simulink model "lab2"  (R2016a)
settings: Solver=FixedStepDiscrete  StartTime=0.0  StopTime=inf  FixedStep=Ts  RelTol=1e-3
values from neighbouring files (symbols this model uses):
  feedback_gain = [0 0 0 0]    [setup_lab2.m]    (also in your_code.m = dlqr(Phi, Gam, Q1, Q2); your_code1.m = dlqr(d_sys.A, d_sys.B, Q1, Q2); your_code2.m = dlqr(Phi, Gam, Q1, Q2); your_code3.m = dlqr(Phi, Gam, Q1, Q2))
  integral_gain = 0    [setup_lab2.m]
undefined symbols (not defined in the file or in its folder): DiscIntNeverNeededParam
libraries: cstblocks x2, MinSegLibrary_M1V4 x2, simulink x1, dspsigops x1
settings Model: SimulationMode=external  ExtModeTrigDuration=2  Creator=Alec  LastModifiedBy=nilsv
settings DataIOCC: LimitDataPoints=on  SaveFormat=Array  SaveOutput=off  SignalLogging=off  DSMLogging=off  VisualizeSimOutput=off  SaveTime=off
settings OptimizationCC: PassReuseOutputArgsThreshold=0  ExpressionDepthLimit=2147483647  MaxStackSize=64
settings DebuggingCC: UnderspecifiedInitializationDetection=Classic  MergeDetectMultiDrivingBlocksExec=none  ParameterTunabilityLossMsg=error  UnconnectedInputMsg=none  UnconnectedOutputMsg=none  StateNameClashWarn=warning
settings HardwareCC: ProdBitPerInt=16  ProdBitPerPointer=16  ProdLargestAtomicFloat=None  ProdWordSize=8  ProdHWDeviceType=Atmel->AVR  UseEmbeddedCoderFeatures=off  UseSimulinkCoderFeatures=off
settings ModelReferenceCC: PropagateSignalLabelsOutOfModel=off
settings RTWCC: SystemTargetFile=ert.tlc  HardwareBoard=Arduino Mega 2560  TLCOptions=-aInlineSetEventsForThisBaseRateFcn=TLC_FALSE -aSuppressMultiTaskScheduler=TLC_FALSE -aRateBasedStepFcn=1  TemplateMakefile=ert_default_tmf  RTWVerbose=off  Toolchain=Arduino AVR v1.6.1  BuildConfiguration=Faster Runs
settings CodeAppCC: ForceParamTrailComments=on  OperatorAnnotations=on  MangleLength=10
settings ERTTargetCC: MultiwordLength=256  ERTCustomFileBanners=off  SupportContinuousTime=on  SupportNonInlinedSFcns=on  SupportVariableSizeSignals=on  ModelStepFunctionPrototypeControlCompliant=off  ExtMode=on  ExtModeTransport=3  ExtModeMexFile=ext_serial_win32_comm_rtt  ExtModeMexArgs=0 '/dev/ttyACM0' 115200  ERTSrcFileBannerTemplate=codertarget_code_template.cgt  ERTHdrFileBannerTemplate=codertarget_code_template.cgt  ERTDataSrcFileTemplate=codertarget_code_template.cgt  ERTDataHdrFileTemplate=codertarget_code_template.cgt
settings ConfigComp: CovEnableCumulative=off  CovSaveSingleToWorkspaceVar=off  CovSaveOutputData=off

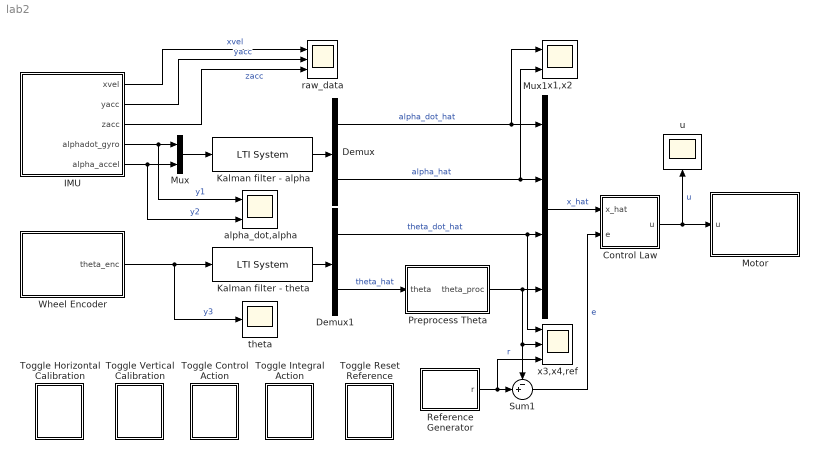
== system lab2 ==
  Control Law : Subsystem
  Demux : Demux  Outputs=2
  Demux1 : Demux  Outputs=2
  IMU : Subsystem
  Kalman filter - alpha : cstblocks/LTI System  sys=imu_kalman  IC=[]
  Kalman filter - theta : cstblocks/LTI System  sys=wheel_kalman  IC=[]
  Motor : Subsystem
  Mux : Mux  Inputs=2
  Mux1 : Mux
  Preprocess Theta : Subsystem
  Reference Generator : Subsystem  mask{amplitude_reference=0}
      mask prompts: amplitude_reference "Amplitude"
      mask DialogControl DescTextVar Prompt: Reference Generator. Please set the amplitude of the reference signal to follow.
      mask Display:
      | y = [-1,-1,-1,-1,-1,-1,-1,-1,-1,-0.6,-0.2,0.2,0.6,1,1,1,1,1,1,1,1,1,1,1,1,1,1,1,1,1,1,0.6,0.2,-0.2,-0.6,-1,-1,-1,-1,-1,-1,-1,-1,-1];
      | x = [-1,-0.96078,-0.92157,-0.88235,-0.84314,-0.80392,-0.76471,-0.72549,-0.68627,-0.56863,-0.52941,-0.4902,-0.45098,-0.33333,-0.29412,-0.2549,-0.21569,-0.17647,-0.13725,-0.098039,-0.058824,-0.019608,0.019608,0.058824,0.098039,0.13725,0.17647,0.21569,0.2549,0.29412,0.33333,0.45098,0.4902,0.52941,0.56863,0.68627,0.72549,0.76471,0.80392,0.84314,0.88235,0.92157,0.96078,1];
      | plot(x, y);
  Sum1 : Sum  Inputs=-+|
  Toggle Control Action : Subsystem  DialogController=hmiCreateDDGDialog  IsWebBlock=on  mask(MWDashboardBlock){webBlockId=64fc8a19-04bc-47ff-b6b8-cd18ab5ec033, webBlockType=toggleswitch, ShowInLibBrowser=on, ShowInitialText=on, HMISrcModelName=lab2}
      mask prompts: webBlockId "WebBlock Id"; webBlockType "WebBlock Type"; HMISrcModelName "Source Model"
      mask Help: helpview([docroot '/mapfiles/simulink.map'], 'hmi_toggle_switch')
      mask Display:
      | if strcmp(get_param(bdroot(gcb),'BlockDiagramType'), 'library')
      |     image([(matlabroot) '/toolbox/simulink/hmi/icons/ToggleSwitch.png']);
      | end
  Toggle Integral Action : Subsystem  DialogController=hmiCreateDDGDialog  IsWebBlock=on  mask(MWDashboardBlock){webBlockId=4f1e93d4-160d-4872-a41a-e243eeba8d4a, webBlockType=toggleswitch, ShowInLibBrowser=on, ShowInitialText=on, HMISrcModelName=lab2}
      mask prompts: webBlockId "WebBlock Id"; webBlockType "WebBlock Type"; HMISrcModelName "Source Model"
      mask Help: helpview([docroot '/mapfiles/simulink.map'], 'hmi_toggle_switch')
      mask Display:
      | if strcmp(get_param(bdroot(gcb),'BlockDiagramType'), 'library')
      |     image([(matlabroot) '/toolbox/simulink/hmi/icons/ToggleSwitch.png']);
      | end
  Toggle Reset Reference : Subsystem  DialogController=hmiCreateDDGDialog  IsWebBlock=on  mask(MWDashboardBlock){webBlockId=51dc4b42-a644-48db-9e68-323c48c3ab41, webBlockType=toggleswitch, ShowInLibBrowser=on, ShowInitialText=on, HMISrcModelName=lab2}
      mask prompts: webBlockId "WebBlock Id"; webBlockType "WebBlock Type"; HMISrcModelName "Source Model"
      mask Help: helpview([docroot '/mapfiles/simulink.map'], 'hmi_toggle_switch')
      mask Display:
      | if strcmp(get_param(bdroot(gcb),'BlockDiagramType'), 'library')
      |     image([(matlabroot) '/toolbox/simulink/hmi/icons/ToggleSwitch.png']);
      | end
  Toggle Horizontal Calibration : Subsystem  DialogController=hmiCreateDDGDialog  IsWebBlock=on  mask(MWDashboardBlock){webBlockId=eadab8c8-cd35-48e9-8b59-a5b0521da82c, webBlockType=toggleswitch, ShowInLibBrowser=on, ShowInitialText=on, HMISrcModelName=lab2}
      mask prompts: webBlockId "WebBlock Id"; webBlockType "WebBlock Type"; HMISrcModelName "Source Model"
      mask Help: helpview([docroot '/mapfiles/simulink.map'], 'hmi_toggle_switch')
      mask Display:
      | if strcmp(get_param(bdroot(gcb),'BlockDiagramType'), 'library')
      |     image([(matlabroot) '/toolbox/simulink/hmi/icons/ToggleSwitch.png']);
      | end
  Toggle Vertical Calibration : Subsystem  DialogController=hmiCreateDDGDialog  IsWebBlock=on  mask(MWDashboardBlock){webBlockId=45f31a6e-857f-48e6-b054-7e32dd315763, webBlockType=toggleswitch, ShowInLibBrowser=on, ShowInitialText=on, HMISrcModelName=lab2}
      mask prompts: webBlockId "WebBlock Id"; webBlockType "WebBlock Type"; HMISrcModelName "Source Model"
      mask Help: helpview([docroot '/mapfiles/simulink.map'], 'hmi_toggle_switch')
      mask Display:
      | if strcmp(get_param(bdroot(gcb),'BlockDiagramType'), 'library')
      |     image([(matlabroot) '/toolbox/simulink/hmi/icons/ToggleSwitch.png']);
      | end
  Wheel Encoder : Subsystem
  alpha_dot,alpha : Scope  NumInputPorts=2
  raw_data : Scope  NumInputPorts=3
  theta : Scope
  u : Scope
  x1,x2 : Scope  NumInputPorts=2
  x3,x4,ref : Scope  NumInputPorts=3
  wires:
  Mux/1 -> Kalman filter - alpha/1
  Demux/2 -> x1,x2/2, Mux1/2  "alpha_hat"
  Demux/1 -> x1,x2/1, Mux1/1  "alpha_dot_hat"
  Mux1/1 -> Control Law/1(x_hat)  "x_hat"
  Wheel Encoder/1(theta_enc) -> theta/1, Kalman filter - theta/1  "y3"
  Demux1/1 -> x3,x4,ref/1, Mux1/3  "theta_dot_hat"
  Demux1/2 -> Preprocess Theta/1(theta)  "theta_hat"
  Kalman filter - theta/1 -> Demux1/1
  Control Law/1(u) -> Motor/1(u), u/1  "u"
  IMU/5(alpha_accel) -> alpha_dot,alpha/2, Mux/2  "y2"
  IMU/4(alphadot_gyro) -> alpha_dot,alpha/1, Mux/1  "y1"
  Reference Generator/1(r) -> Sum1/2, x3,x4,ref/3  "r"
  Preprocess Theta/1(theta_proc) -> Mux1/4, Sum1/1, x3,x4,ref/2
  Kalman filter - alpha/1 -> Demux/1
  Sum1/1 -> Control Law/2(e)  "e"
  IMU/1(xvel) -> raw_data/1  "xvel"
  IMU/3(zacc) -> raw_data/3  "zacc"
  IMU/2(yacc) -> raw_data/2  "yacc"

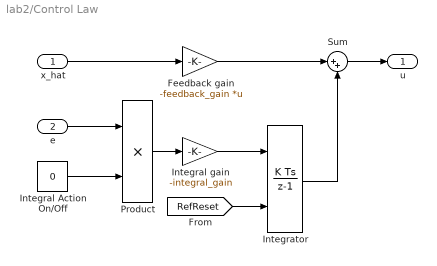
== system lab2/Control Law ==
  x_hat : Inport
  e : Inport  Port=2
  Feedback gain : Gain  Gain=-feedback_gain  Multiplication=Matrix(K*u)
  Integral Action On/Off : Constant  Value=0
  Integral gain : Gain  Gain=-integral_gain
  Integrator : DiscreteIntegrator  gainval=1  ExternalReset=either  InitialConditionSetting=State (most efficient)  SampleTime=-1  ICPrevOutput=DiscIntNeverNeededParam  ICPrevScaledInput=DiscIntNeverNeededParam
  Product : Product
  Sum : Sum  Inputs=|++
  u : Outport
  wires:
  Integral gain/1 -> Integrator/1
  x_hat/1 -> Feedback gain/1
  Feedback gain/1 -> Sum/1
  Sum/1 -> u/1
  Product/1 -> Integral gain/1
  e/1 -> Product/1
  Integral Action On/Off/1 -> Product/2
  Integrator/1 -> Sum/2
  [RefReset] -> Integrator/2

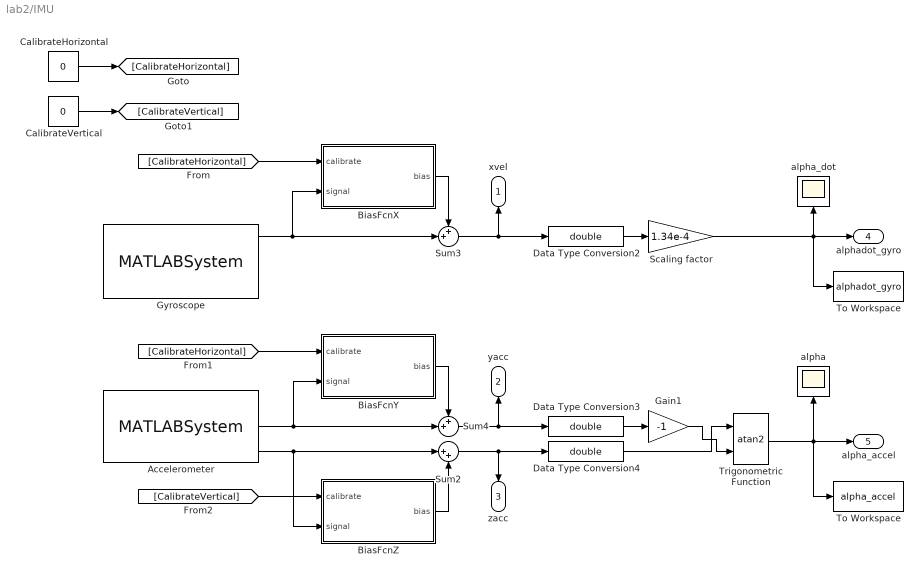
== system lab2/IMU ==
  " To Workspace " : ToWorkspace  VariableName=alpha_accel  SampleTime=-1
      settings: Save2DSignal=2-D array (concatenate along first dimension)
  Accelerometer : MATLABSystem  System=soMPU6050Accel  SimulateUsing=Code generation
      mask Type: soMPU6050Accel
      mask Display:
      | disp('soMPU6050Accel');
      | port_label('output',1,'xaccel');
      | port_label('output',2,'yaccel');
      | port_label('output',3,'zaccel');
  BiasFcnX : MATLAB Function  TreatAsAtomicUnit=on
  BiasFcnY : MATLAB Function  TreatAsAtomicUnit=on
  BiasFcnZ : MATLAB Function  TreatAsAtomicUnit=on
  CalibrateHorizontal : Constant  Value=0  OutDataTypeStr=boolean
  CalibrateVertical : Constant  Value=0  OutDataTypeStr=boolean
  Data Type Conversion2 : DataTypeConversion  OutDataTypeStr=double
  Data Type Conversion3 : DataTypeConversion  OutDataTypeStr=double
  Data Type Conversion4 : DataTypeConversion  OutDataTypeStr=double
  Gain1 : Gain  Gain=-1
  Gyroscope : MATLABSystem  System=soMPU6050Gyro  DLPFmode=0
      mask Type: soMPU6050Gyro
      mask Display:
      | disp('soMPU6050Gyro');
      | port_label('output',1,'xvel');
      | port_label('output',2,'yvel');
      | port_label('output',3,'zvel');
  Scaling factor : Gain  Gain=1.34e-4
  Sum2 : Sum  Inputs=|++
  Sum3 : Sum  Inputs=++|
  Sum4 : Sum  Inputs=++|
  To Workspace : ToWorkspace  VariableName=alphadot_gyro  SampleTime=-1
      settings: Save2DSignal=2-D array (concatenate along first dimension)
  Trigonometric Function : Trigonometry  Operator=atan2
  alpha : Scope
  alpha_dot : Scope
  xvel : Outport
  yacc : Outport  Port=2
  zacc : Outport  Port=3
  alphadot_gyro : Outport  Port=4
  alpha_accel : Outport  Port=5
  wires:
  Gyroscope/1 -> BiasFcnX/2(signal), Sum3/2
  Sum3/1 -> xvel/1, Data Type Conversion2/1
  Data Type Conversion2/1 -> Scaling factor/1
  Scaling factor/1 -> alpha_dot/1, alphadot_gyro/1, To Workspace/1
  BiasFcnX/1(bias) -> Sum3/1
  Sum4/1 -> yacc/1, Data Type Conversion3/1
  Sum2/1 -> zacc/1, Data Type Conversion4/1
  Data Type Conversion3/1 -> Gain1/1
  Data Type Conversion4/1 -> Trigonometric Function/1
  Gain1/1 -> Trigonometric Function/2
  Trigonometric Function/1 -> alpha/1, " To Workspace "/1, alpha_accel/1
  [CalibrateHorizontal] -> BiasFcnX/1(calibrate)
  Accelerometer/2 -> BiasFcnY/2(signal), Sum4/2
  BiasFcnY/1(bias) -> Sum4/1
  [CalibrateHorizontal] -> BiasFcnY/1(calibrate)
  Accelerometer/3 -> BiasFcnZ/2(signal), Sum2/1
  BiasFcnZ/1(bias) -> Sum2/2
  [CalibrateVertical] -> BiasFcnZ/1(calibrate)
  CalibrateHorizontal/1 -> [CalibrateHorizontal]
  CalibrateVertical/1 -> [CalibrateVertical]

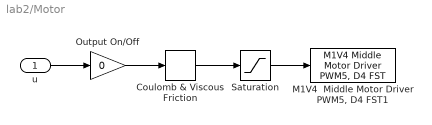
== system lab2/Motor ==
  u : Inport
  Coulomb & Viscous Friction : simulink/Discontinuities/Coulomb & Viscous Friction  offset=0.25  gain=1
  "M1V4  Middle Motor Driver PWM5, D4 FST1" : MinSegLibrary_M1V4/M1V4  Middle Motor Driver PWM5, D4 FST  Vsupply=3.25
  Output On/Off : Gain  Gain=0
  Saturation : Saturate  UpperLimit=3.25  LowerLimit=-3.25
  wires:
  u/1 -> Output On/Off/1
  Coulomb & Viscous Friction/1 -> Saturation/1
  Saturation/1 -> "M1V4  Middle Motor Driver PWM5, D4 FST1"/1
  Output On/Off/1 -> Coulomb & Viscous Friction/1

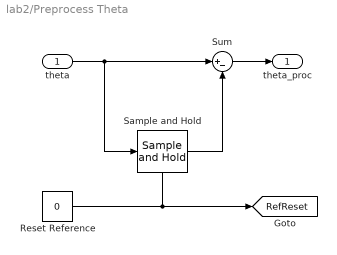
== system lab2/Preprocess Theta ==
  theta : Inport
  Reset Reference : Constant  Value=0
  Sample and Hold : dspsigops/Sample and Hold  trig=Either edge  initCond=0  latchinput=off
  Sum : Sum  Inputs=|+-
  theta_proc : Outport
  tag scope: RefReset=global
  wires:
  theta/1 -> Sample and Hold/1, Sum/1
  Sum/1 -> theta_proc/1
  Reset Reference/1 -> [RefReset], Sample and Hold/Trigger
  Sample and Hold/1 -> Sum/2

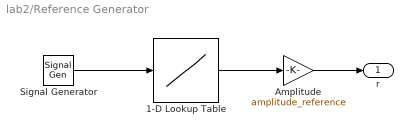
== system lab2/Reference Generator ==
  1-D Lookup Table : Lookup_n-D  NumberOfTableDimensions=1  BreakpointsForDimension1=[-1,-0.96078,-0.92157,-0.88235,-0.84314,-0.80392,-0.76471,-0.72549,-0.68627,-0.56863,-0.52941,-0.4902,-0.45098,-0.33333,-0.29412,-0.2549,-0.21569,-0.17647,-0.13725,-0.098039,-0.058824,-0.019608,0.019608,0.058824,0.098039,0.13725,0.17647,0.21569,0.2549,0.29412,0.33333,0.45098,0.4902,0.52941,0.56863,0.68627,0.72549,0.76471,0.80392,0.84314,0.88235,0.92157,0.96078,1]  Table=[-1, -1, -1, -1, -1, -1, -1, -1, -1, -0.6, -0.2, 0.2, 0.6, 1, 1, 1, 1, 1, 1, 1, 1, 1, 1, 1, 1, 1, 1, 1, 1, 1, 1, 0.6, 0.2, -0.2, -0.6, -1, -1, -1, -1, -1, -1, -1, -1, -1]  InterpMethod=Cubic spline  InternalRulePriority=Speed  RndMeth=Simplest  InputSameDT=on
  Amplitude : Gain  Gain=amplitude_reference
  Signal Generator : SignalGenerator  WaveForm=sawtooth  Frequency=0.025
  r : Outport
  wires:
  1-D Lookup Table/1 -> Amplitude/1
  Signal Generator/1 -> 1-D Lookup Table/1
  Amplitude/1 -> r/1

== system lab2/Toggle Control Action ==

== system lab2/Toggle Integral Action ==

== system lab2/Toggle Reset Reference ==

== system lab2/Toggle Horizontal Calibration ==

== system lab2/Toggle Vertical Calibration ==

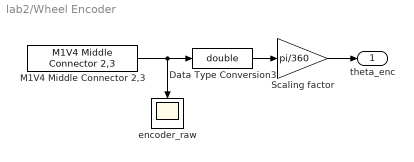
== system lab2/Wheel Encoder ==
  Data Type Conversion3 : DataTypeConversion  OutDataTypeStr=double
  M1V4 Middle Connector 2,3 : MinSegLibrary_M1V4/M1V4 Middle Connector 2,3  Encoder=0  PinA=3  PinB=2
  Scaling factor : Gain  Gain=pi/360
  encoder_raw : Scope
  theta_enc : Outport
  wires:
  Data Type Conversion3/1 -> Scaling factor/1
  Scaling factor/1 -> theta_enc/1
  M1V4 Middle Connector 2,3/1 -> encoder_raw/1, Data Type Conversion3/1

== matlab function lab2/IMU/BiasFcnY ==
  data: calibrate input; bias output; signal input
function bias = offset_fcn(calibrate, signal)
%#codegen

% Set all the persistent variables
%   offset  = the offset to output
%   memory  = the stored signal
%   itr     = the iterator keeping track of where we are in the memory
persistent offset memory itr max_itr finished;

if isempty(memory)
    max_itr  = 150;
    itr      = 1;
    memory   = zeros(max_itr, 1);
    offset   = 0;
    finished = 0;
end

% If we are currently calibrating the offset
if calibrate && ~finished
    memory(itr) = signal;
    offset = -mean(memory);
    itr = itr + 1;
    if itr > max_itr
        finished = 1;
    end
elseif ~calibrate
    finished = 0;
    itr = 1;
end

bias = offset;
end

== matlab function lab2/IMU/BiasFcnX ==
  data: calibrate input; bias output; signal input
function bias = offset_fcn(calibrate, signal)
%#codegen

% Set all the persistent variables
%   offset  = the offset to output
%   memory  = the stored signal
%   itr     = the iterator keeping track of where we are in the memory
persistent offset memory itr max_itr finished;

if isempty(memory)
    max_itr  = 100;
    itr      = 1;
    memory   = zeros(max_itr, 1);
    offset   = 0;
    finished = 0;
end

% If we are currently calibrating the offset
if calibrate && ~finished
    memory(itr) = signal;
    offset = -mean(memory);
    itr = itr + 1;
    if itr > max_itr
        finished = 1;
    end
elseif ~calibrate
    finished = 0;
    itr = 1;
end

bias = offset;
end

== matlab function lab2/IMU/BiasFcnZ ==
  data: calibrate input; bias output; signal input
function bias = offset_fcn(calibrate, signal)
%#codegen

% Set all the persistent variables
%   offset  = the offset to output
%   memory  = the stored signal
%   itr     = the iterator keeping track of where we are in the memory
persistent offset memory itr max_itr finished;

if isempty(memory)
    max_itr  = 200;
    itr      = 1;
    memory   = zeros(max_itr, 1);
    offset   = 0;
    finished = 0;
end

% If we are currently calibrating the offset
if calibrate && ~finished
    memory(itr) = signal;
    offset = -mean(memory);
    itr = itr + 1;
    if itr > max_itr
        finished = 1;
    end
elseif ~calibrate
    finished = 0;
    itr = 1;
end

bias = offset;
end
